simulink library "halout"  (R2021b)
settings: Solver=VariableStepAuto  StartTime=0.0  StopTime=10.0  RelTol=1e-3
undefined symbols (not defined in the file): C_TASK_5MS_S, KHAL_CAN1TxReq_flg, KHAL_CAN2TxReq_flg, KHAL_CAN3TxReq_flg, KHAL_CAN4TxReq_flg, KHAL_CAN5TxReq_flg, KHAL_CAN6TxReq_flg, KHAL_CAN7TxReq_flg, TRUE
libraries: FVT_lib x65, simulink x6
(part 2 of 6)

== system halout/HAL_OUT/CAN1/FD1_C50_0_0x18F00503 ==
  BSCP_outputs : Inport  OutDataTypeStr=Bus: BSCP_outputs
  BOUTP_outputs : Inport  Port=2  OutDataTypeStr=Bus: BOUTP_outputs
  ActDriveDirect : Subsystem
  Ground : Ground
  bus_creator : BusCreator  Inputs=1  OutDataTypeStr=Bus: DT_CAN1_SG_FD1_C50_0  NonVirtualBus=on
  FD1_C50_0 : Outport
  wires:
  BSCP_outputs/1 -> [BSCP_outputs]
  BOUTP_outputs/1 -> [BOUTP_outputs]
  [CAN1_ActDriveDirect] -> bus_creator/1  "CAN1_ActDriveDirect"
  bus_creator/1 -> FD1_C50_0/1
  ActDriveDirect/1(CAN1_ActDriveDirect) -> [CAN1_ActDriveDirect]
  Ground/1 -> ActDriveDirect/1(ActDriveDirect)

== system halout/HAL_OUT/CAN1/FD1_C50_1_0xCF00300 ==
  BSCP_outputs : Inport  OutDataTypeStr=Bus: BSCP_outputs
  BOUTP_outputs : Inport  Port=2  OutDataTypeStr=Bus: BOUTP_outputs
  AccPedal1LowSW : Subsystem
  AccPedalPos1 : Subsystem
  EEC2MSGCS : Subsystem
  EEC2MSGCnt : Subsystem
  Ground{,1..3} (4 alike) : Ground
  bus_creator : BusCreator  Inputs=4  OutDataTypeStr=Bus: DT_CAN1_SG_FD1_C50_1  NonVirtualBus=on
  FD1_C50_1 : Outport
  wires:
  BSCP_outputs/1 -> [BSCP_outputs]
  BOUTP_outputs/1 -> [BOUTP_outputs]
  [CAN1_AccPedal1LowSW] -> bus_creator/1  "CAN1_AccPedal1LowSW"
  [CAN1_AccPedalPos1] -> bus_creator/2  "CAN1_AccPedalPos1"
  [CAN1_EEC2MSGCS] -> bus_creator/3  "CAN1_EEC2MSGCS"
  [CAN1_EEC2MSGCnt] -> bus_creator/4  "CAN1_EEC2MSGCnt"
  bus_creator/1 -> FD1_C50_1/1
  AccPedal1LowSW/1(CAN1_AccPedal1LowSW) -> [CAN1_AccPedal1LowSW]
  AccPedalPos1/1(CAN1_AccPedalPos1) -> [CAN1_AccPedalPos1]
  EEC2MSGCS/1(CAN1_EEC2MSGCS) -> [CAN1_EEC2MSGCS]
  EEC2MSGCnt/1(CAN1_EEC2MSGCnt) -> [CAN1_EEC2MSGCnt]
  Ground/1 -> AccPedal1LowSW/1(AccPedal1LowSW)
  Ground1/1 -> AccPedalPos1/1(AccPedalPos1)
  Ground2/1 -> EEC2MSGCS/1(EEC2MSGCS)
  Ground3/1 -> EEC2MSGCnt/1(EEC2MSGCnt)

== system halout/HAL_OUT/CAN1/FD1_C80_0_0x18F00203 ==
  BSCP_outputs : Inport  OutDataTypeStr=Bus: BSCP_outputs
  BOUTP_outputs : Inport  Port=2  OutDataTypeStr=Bus: BOUTP_outputs
  DLEngaged : Subsystem
  ShiftPgs : Subsystem
  bus_creator : BusCreator  Inputs=2  OutDataTypeStr=Bus: DT_CAN1_SG_FD1_C80_0  NonVirtualBus=on
  bus_selector : BusSelector  OutputSignals=VOUTP_DrivelineRelease_enum
  bus_selector1 : BusSelector  OutputSignals=VOUTP_ETC1ShiftrPgs_enum
  FD1_C80_0 : Outport
  wires:
  BSCP_outputs/1 -> [BSCP_outputs]
  BOUTP_outputs/1 -> [BOUTP_outputs]
  [CAN1_DLEngaged] -> bus_creator/1  "CAN1_DLEngaged"
  [CAN1_ShiftPgs] -> bus_creator/2  "CAN1_ShiftPgs"
  bus_creator/1 -> FD1_C80_0/1
  DLEngaged/1(CAN1_DLEngaged) -> [CAN1_DLEngaged]
  ShiftPgs/1(CAN1_ShiftPgs) -> [CAN1_ShiftPgs]
  bus_selector/1 -> DLEngaged/1(DLEngaged)  "<VOUTP_DrivelineRelease_enum>"
  [BOUTP_outputs] -> bus_selector/1
  bus_selector1/1 -> ShiftPgs/1(ShiftPgs)  "<VOUTP_ETC1ShiftrPgs_enum>"
  [BOUTP_outputs] -> bus_selector1/1

== system halout/HAL_OUT/CAN1/FD1_CE100_0_0x18EBFFEF ==
  BSCP_outputs : Inport  OutDataTypeStr=Bus: BSCP_outputs
  BOUTP_outputs : Inport  Port=2  OutDataTypeStr=Bus: BOUTP_outputs
  CFGEM1DT0 : Subsystem
  CFGEM1DT1 : Subsystem
  CFGEM1DT2 : Subsystem
  CFGEM1DT3 : Subsystem
  CFGEM1DT4 : Subsystem
  CFGEM1DT5 : Subsystem
  CFGEM1DT6 : Subsystem
  CFGEM1DT7 : Subsystem
  bus_creator : BusCreator  Inputs=8  OutDataTypeStr=Bus: DT_CAN1_SG_FD1_CE100_0  NonVirtualBus=on
  bus_selector : BusSelector  OutputSignals=VOUTP_DTbyte0_raw
  bus_selector1 : BusSelector  OutputSignals=VOUTP_DTbyte1_raw
  bus_selector2 : BusSelector  OutputSignals=VOUTP_DTbyte2_raw
  bus_selector3 : BusSelector  OutputSignals=VOUTP_DTbyte3_raw
  bus_selector4 : BusSelector  OutputSignals=VOUTP_DTbyte4_raw
  bus_selector5 : BusSelector  OutputSignals=VOUTP_DTbyte5_raw
  bus_selector6 : BusSelector  OutputSignals=VOUTP_DTbyte6_raw
  bus_selector7 : BusSelector  OutputSignals=VOUTP_DTbyte7_raw
  FD1_CE100_0 : Outport
  wires:
  BSCP_outputs/1 -> [BSCP_outputs]
  BOUTP_outputs/1 -> [BOUTP_outputs]
  [CAN1_CFGEM1DT0] -> bus_creator/1  "CAN1_CFGEM1DT0"
  [CAN1_CFGEM1DT1] -> bus_creator/2  "CAN1_CFGEM1DT1"
  [CAN1_CFGEM1DT2] -> bus_creator/3  "CAN1_CFGEM1DT2"
  [CAN1_CFGEM1DT3] -> bus_creator/4  "CAN1_CFGEM1DT3"
  [CAN1_CFGEM1DT4] -> bus_creator/5  "CAN1_CFGEM1DT4"
  [CAN1_CFGEM1DT5] -> bus_creator/6  "CAN1_CFGEM1DT5"
  [CAN1_CFGEM1DT6] -> bus_creator/7  "CAN1_CFGEM1DT6"
  [CAN1_CFGEM1DT7] -> bus_creator/8  "CAN1_CFGEM1DT7"
  bus_creator/1 -> FD1_CE100_0/1
  CFGEM1DT0/1(CAN1_CFGEM1DT0) -> [CAN1_CFGEM1DT0]
  CFGEM1DT1/1(CAN1_CFGEM1DT1) -> [CAN1_CFGEM1DT1]
  CFGEM1DT2/1(CAN1_CFGEM1DT2) -> [CAN1_CFGEM1DT2]
  CFGEM1DT3/1(CAN1_CFGEM1DT3) -> [CAN1_CFGEM1DT3]
  CFGEM1DT4/1(CAN1_CFGEM1DT4) -> [CAN1_CFGEM1DT4]
  CFGEM1DT5/1(CAN1_CFGEM1DT5) -> [CAN1_CFGEM1DT5]
  CFGEM1DT6/1(CAN1_CFGEM1DT6) -> [CAN1_CFGEM1DT6]
  CFGEM1DT7/1(CAN1_CFGEM1DT7) -> [CAN1_CFGEM1DT7]
  bus_selector/1 -> CFGEM1DT0/1(CFGEM1DT0)  "<VOUTP_DTbyte0_raw>"
  [BOUTP_outputs] -> bus_selector/1
  bus_selector1/1 -> CFGEM1DT1/1(CFGEM1DT1)  "<VOUTP_DTbyte1_raw>"
  [BOUTP_outputs] -> bus_selector1/1
  bus_selector2/1 -> CFGEM1DT2/1(CFGEM1DT2)  "<VOUTP_DTbyte2_raw>"
  [BOUTP_outputs] -> bus_selector2/1
  bus_selector3/1 -> CFGEM1DT3/1(CFGEM1DT3)  "<VOUTP_DTbyte3_raw>"
  [BOUTP_outputs] -> bus_selector3/1
  bus_selector4/1 -> CFGEM1DT4/1(CFGEM1DT4)  "<VOUTP_DTbyte4_raw>"
  [BOUTP_outputs] -> bus_selector4/1
  bus_selector5/1 -> CFGEM1DT5/1(CFGEM1DT5)  "<VOUTP_DTbyte5_raw>"
  [BOUTP_outputs] -> bus_selector5/1
  bus_selector6/1 -> CFGEM1DT6/1(CFGEM1DT6)  "<VOUTP_DTbyte6_raw>"
  [BOUTP_outputs] -> bus_selector6/1
  bus_selector7/1 -> CFGEM1DT7/1(CFGEM1DT7)  "<VOUTP_DTbyte7_raw>"
  [BOUTP_outputs] -> bus_selector7/1

== system halout/HAL_OUT/CAN1/FD1_CE100_1_0x18ECFFEF ==
  BSCP_outputs : Inport  OutDataTypeStr=Bus: BSCP_outputs
  BOUTP_outputs : Inport  Port=2  OutDataTypeStr=Bus: BOUTP_outputs
  CFGEM1BAMPGN : Subsystem
  CFGEM1BAMRsv : Subsystem
  CFGEM1BAMTNum : Subsystem
  CFGEM1BAMTSize : Subsystem
  CFGEM1Ctrl : Subsystem
  bus_creator : BusCreator  Inputs=5  OutDataTypeStr=Bus: DT_CAN1_SG_FD1_CE100_1  NonVirtualBus=on
  bus_selector : BusSelector  OutputSignals=VOUTP_CFGEM1BAMPGN_raw
  bus_selector1 : BusSelector  OutputSignals=VOUTP_CFGEM1BAMRsv_raw
  bus_selector2 : BusSelector  OutputSignals=VOUTP_CFGEM1BAMTNum_raw
  bus_selector3 : BusSelector  OutputSignals=VOUTP_CFGEM1BAMTSize_raw
  bus_selector4 : BusSelector  OutputSignals=VOUTP_CFGEM1Ctrl_raw
  FD1_CE100_1 : Outport
  wires:
  BSCP_outputs/1 -> [BSCP_outputs]
  BOUTP_outputs/1 -> [BOUTP_outputs]
  [CAN1_CFGEM1BAMPGN] -> bus_creator/1  "CAN1_CFGEM1BAMPGN"
  [CAN1_CFGEM1BAMRsv] -> bus_creator/2  "CAN1_CFGEM1BAMRsv"
  [CAN1_CFGEM1BAMTNum] -> bus_creator/3  "CAN1_CFGEM1BAMTNum"
  [CAN1_CFGEM1BAMTSize] -> bus_creator/4  "CAN1_CFGEM1BAMTSize"
  [CAN1_CFGEM1Ctrl] -> bus_creator/5  "CAN1_CFGEM1Ctrl"
  bus_creator/1 -> FD1_CE100_1/1
  CFGEM1BAMPGN/1(CAN1_CFGEM1BAMPGN) -> [CAN1_CFGEM1BAMPGN]
  CFGEM1BAMRsv/1(CAN1_CFGEM1BAMRsv) -> [CAN1_CFGEM1BAMRsv]
  CFGEM1BAMTNum/1(CAN1_CFGEM1BAMTNum) -> [CAN1_CFGEM1BAMTNum]
  CFGEM1BAMTSize/1(CAN1_CFGEM1BAMTSize) -> [CAN1_CFGEM1BAMTSize]
  CFGEM1Ctrl/1(CAN1_CFGEM1Ctrl) -> [CAN1_CFGEM1Ctrl]
  bus_selector/1 -> CFGEM1BAMPGN/1(CFGEM1BAMPGN)  "<VOUTP_CFGEM1BAMPGN_raw>"
  [BOUTP_outputs] -> bus_selector/1
  bus_selector1/1 -> CFGEM1BAMRsv/1(CFGEM1BAMRsv)  "<VOUTP_CFGEM1BAMRsv_raw>"
  [BOUTP_outputs] -> bus_selector1/1
  bus_selector2/1 -> CFGEM1BAMTNum/1(CFGEM1BAMTNum)  "<VOUTP_CFGEM1BAMTNum_raw>"
  [BOUTP_outputs] -> bus_selector2/1
  bus_selector3/1 -> CFGEM1BAMTSize/1(CFGEM1BAMTSize)  "<VOUTP_CFGEM1BAMTSize_raw>"
  [BOUTP_outputs] -> bus_selector3/1
  bus_selector4/1 -> CFGEM1Ctrl/1(CFGEM1Ctrl)  "<VOUTP_CFGEM1Ctrl_raw>"
  [BOUTP_outputs] -> bus_selector4/1

== system halout/HAL_OUT/CAN1/FD1_CE100_2_0x18FA05B9 ==
  BSCP_outputs : Inport  OutDataTypeStr=Bus: BSCP_outputs
  BOUTP_outputs : Inport  Port=2  OutDataTypeStr=Bus: BOUTP_outputs
  FDCBCMDVRSignalLCmd : Subsystem
  FDCBCMDVRSignalRCmd : Subsystem
  FDCBCMLTurnLpCmd : Subsystem
  FDCBCMRTurnLpCmd : Subsystem
  bus_creator : BusCreator  Inputs=4  OutDataTypeStr=Bus: DT_CAN1_SG_FD1_CE100_2  NonVirtualBus=on
  bus_selector : BusSelector  OutputSignals=VOUTP_FDCBCMDVRSignalLCmd_flg
  bus_selector1 : BusSelector  OutputSignals=VOUTP_FDCBCMDVRSignalRCmd_flg
  bus_selector2 : BusSelector  OutputSignals=VOUTP_FDCBCMLTurnLpCmd_flg
  bus_selector3 : BusSelector  OutputSignals=VOUTP_FDCBCMRTurnLpCmd_flg
  FD1_CE100_2 : Outport
  wires:
  BSCP_outputs/1 -> [BSCP_outputs]
  BOUTP_outputs/1 -> [BOUTP_outputs]
  [CAN1_FDC_BCM_DVRSignalL_Cmd] -> bus_creator/1  "CAN1_FDC_BCM_DVRSignalL_Cmd"
  [CAN1_FDC_BCM_DVRSignalR_Cmd] -> bus_creator/2  "CAN1_FDC_BCM_DVRSignalR_Cmd"
  [CAN1_FDC_BCM_LTurnLp_Cmd] -> bus_creator/3  "CAN1_FDC_BCM_LTurnLp_Cmd"
  [CAN1_FDC_BCM_RTurnLp_Cmd] -> bus_creator/4  "CAN1_FDC_BCM_RTurnLp_Cmd"
  bus_creator/1 -> FD1_CE100_2/1
  FDCBCMDVRSignalLCmd/1(CAN1_FDC_BCM_DVRSignalL_Cmd) -> [CAN1_FDC_BCM_DVRSignalL_Cmd]
  FDCBCMDVRSignalRCmd/1(CAN1_FDC_BCM_DVRSignalR_Cmd) -> [CAN1_FDC_BCM_DVRSignalR_Cmd]
  FDCBCMLTurnLpCmd/1(CAN1_FDC_BCM_LTurnLp_Cmd) -> [CAN1_FDC_BCM_LTurnLp_Cmd]
  FDCBCMRTurnLpCmd/1(CAN1_FDC_BCM_RTurnLp_Cmd) -> [CAN1_FDC_BCM_RTurnLp_Cmd]
  bus_selector/1 -> FDCBCMDVRSignalLCmd/1(FDCBCMDVRSignalLCmd)  "<VOUTP_FDCBCMDVRSignalLCmd_flg>"
  [BOUTP_outputs] -> bus_selector/1
  bus_selector1/1 -> FDCBCMDVRSignalRCmd/1(FDCBCMDVRSignalRCmd)  "<VOUTP_FDCBCMDVRSignalRCmd_flg>"
  [BOUTP_outputs] -> bus_selector1/1
  bus_selector2/1 -> FDCBCMLTurnLpCmd/1(FDCBCMLTurnLpCmd)  "<VOUTP_FDCBCMLTurnLpCmd_flg>"
  [BOUTP_outputs] -> bus_selector2/1
  bus_selector3/1 -> FDCBCMRTurnLpCmd/1(FDCBCMRTurnLpCmd)  "<VOUTP_FDCBCMRTurnLpCmd_flg>"
  [BOUTP_outputs] -> bus_selector3/1

== system halout/HAL_OUT/CAN2/FD2_C1000_0_0x20E ==
  BSCP_outputs : Inport  OutDataTypeStr=Bus: BSCP_outputs
  BOUTP_outputs : Inport  Port=2  OutDataTypeStr=Bus: BOUTP_outputs
  VCUVehAcclLimit : Subsystem
  VCUVehSpdlimit : Subsystem
  bus_creator : BusCreator  Inputs=2  OutDataTypeStr=Bus: DT_CAN2_SG_FD2_C1000_0  NonVirtualBus=on
  bus_selector : BusSelector  OutputSignals=VOUTP_VehAcclLimitTG_mps2
  bus_selector1 : BusSelector  OutputSignals=VOUTP_VehSpdLimitTG_kph
  FD2_C1000_0 : Outport
  wires:
  BSCP_outputs/1 -> [BSCP_outputs]
  BOUTP_outputs/1 -> [BOUTP_outputs]
  [CAN2_VCUVehAcclLimit] -> bus_creator/1  "CAN2_VCUVehAcclLimit"
  [CAN2_VCUVehSpdlimit] -> bus_creator/2  "CAN2_VCUVehSpdlimit"
  bus_creator/1 -> FD2_C1000_0/1
  VCUVehAcclLimit/1(CAN2_VCUVehAcclLimit) -> [CAN2_VCUVehAcclLimit]
  VCUVehSpdlimit/1(CAN2_VCUVehSpdlimit) -> [CAN2_VCUVehSpdlimit]
  bus_selector/1 -> VCUVehAcclLimit/1(VCUVehAcclLimit)  "<VOUTP_VehAcclLimitTG_mps2>"
  [BOUTP_outputs] -> bus_selector/1
  bus_selector1/1 -> VCUVehSpdlimit/1(VCUVehSpdlimit)  "<VOUTP_VehSpdLimitTG_kph>"
  [BOUTP_outputs] -> bus_selector1/1

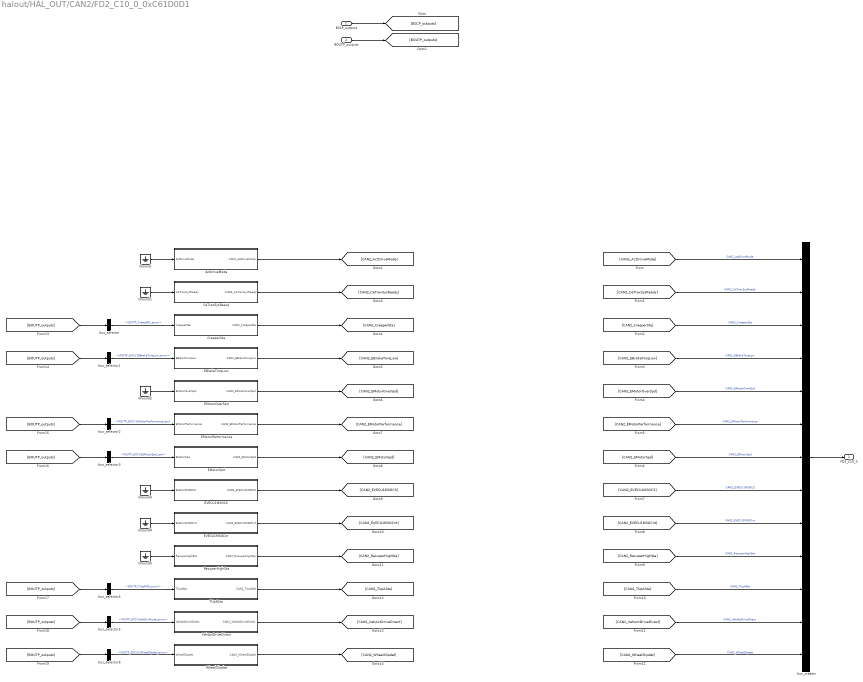
== system halout/HAL_OUT/CAN2/FD2_C10_0_0xC61D0D1 ==
  BSCP_outputs : Inport  OutDataTypeStr=Bus: BSCP_outputs
  BOUTP_outputs : Inport  Port=2  OutDataTypeStr=Bus: BOUTP_outputs
  ActDriveMode : Subsystem
  CeTraxSysReady : Subsystem
  CreeperSta : Subsystem
  EBrakeTorqLow : Subsystem
  EMotorOverSpd : Subsystem
  EMotorPerformance : Subsystem
  EMotorSpd : Subsystem
  EVECU1MSGCS : Subsystem
  EVECU1MSGCnt : Subsystem
  Ground{,1..5} (6 alike) : Ground
  RecuperHighSta : Subsystem
  TUpASta : Subsystem
  VehActDriveDirect : Subsystem
  WheelSlipdet : Subsystem
  bus_creator : BusCreator  Inputs=13  OutDataTypeStr=Bus: DT_CAN2_SG_FD2_C10_0  NonVirtualBus=on
  bus_selector : BusSelector  OutputSignals=VOUTP_CreepIND_enum
  bus_selector1 : BusSelector  OutputSignals=VOUTP_EVCU1EBrakeTorqLow_enum
  bus_selector2 : BusSelector  OutputSignals=VOUTP_EVCU1EMotorPerformance_pct
  bus_selector3 : BusSelector  OutputSignals=VOUTP_EVCU1EMotorSpd_rpm
  bus_selector4 : BusSelector  OutputSignals=VOUTP_TUpAIND_enum
  bus_selector5 : BusSelector  OutputSignals=VOUTP_EVCU1ActDrvMode_enum
  bus_selector6 : BusSelector  OutputSignals=VOUTP_EVCU1WheelSlipdet_enum
  FD2_C10_0 : Outport
  wires:
  BSCP_outputs/1 -> [BSCP_outputs]
  BOUTP_outputs/1 -> [BOUTP_outputs]
  [CAN2_ActDriveMode] -> bus_creator/1  "CAN2_ActDriveMode"
  [CAN2_CeTraxSysReady] -> bus_creator/2  "CAN2_CeTraxSysReady"
  [CAN2_CreeperSta] -> bus_creator/3  "CAN2_CreeperSta"
  [CAN2_EBrakeTorqLow] -> bus_creator/4  "CAN2_EBrakeTorqLow"
  [CAN2_EMotorOverSpd] -> bus_creator/5  "CAN2_EMotorOverSpd"
  [CAN2_EMotorPerformance] -> bus_creator/6  "CAN2_EMotorPerformance"
  [CAN2_EMotorSpd] -> bus_creator/7  "CAN2_EMotorSpd"
  [CAN2_EVECU1MSGCS] -> bus_creator/8  "CAN2_EVECU1MSGCS"
  [CAN2_EVECU1MSGCnt] -> bus_creator/9  "CAN2_EVECU1MSGCnt"
  [CAN2_RecuperHighSta] -> bus_creator/10  "CAN2_RecuperHighSta"
  [CAN2_TUpASta] -> bus_creator/11  "CAN2_TUpASta"
  [CAN2_VehActDriveDirect] -> bus_creator/12  "CAN2_VehActDriveDirect"
  [CAN2_WheelSlipdet] -> bus_creator/13  "CAN2_WheelSlipdet"
  bus_creator/1 -> FD2_C10_0/1
  ActDriveMode/1(CAN2_ActDriveMode) -> [CAN2_ActDriveMode]
  CeTraxSysReady/1(CAN2_CeTraxSysReady) -> [CAN2_CeTraxSysReady]
  CreeperSta/1(CAN2_CreeperSta) -> [CAN2_CreeperSta]
  EBrakeTorqLow/1(CAN2_EBrakeTorqLow) -> [CAN2_EBrakeTorqLow]
  EMotorOverSpd/1(CAN2_EMotorOverSpd) -> [CAN2_EMotorOverSpd]
  EMotorPerformance/1(CAN2_EMotorPerformance) -> [CAN2_EMotorPerformance]
  EMotorSpd/1(CAN2_EMotorSpd) -> [CAN2_EMotorSpd]
  EVECU1MSGCS/1(CAN2_EVECU1MSGCS) -> [CAN2_EVECU1MSGCS]
  EVECU1MSGCnt/1(CAN2_EVECU1MSGCnt) -> [CAN2_EVECU1MSGCnt]
  RecuperHighSta/1(CAN2_RecuperHighSta) -> [CAN2_RecuperHighSta]
  TUpASta/1(CAN2_TUpASta) -> [CAN2_TUpASta]
  VehActDriveDirect/1(CAN2_VehActDriveDirect) -> [CAN2_VehActDriveDirect]
  WheelSlipdet/1(CAN2_WheelSlipdet) -> [CAN2_WheelSlipdet]
  Ground/1 -> ActDriveMode/1(ActDriveMode)
  Ground1/1 -> CeTraxSysReady/1(CeTraxSysReady)
  bus_selector/1 -> CreeperSta/1(CreeperSta)  "<VOUTP_CreepIND_enum>"
  [BOUTP_outputs] -> bus_selector/1
  bus_selector1/1 -> EBrakeTorqLow/1(EBrakeTorqLow)  "<VOUTP_EVCU1EBrakeTorqLow_enum>"
  [BOUTP_outputs] -> bus_selector1/1
  Ground2/1 -> EMotorOverSpd/1(EMotorOverSpd)
  bus_selector2/1 -> EMotorPerformance/1(EMotorPerformance)  "<VOUTP_EVCU1EMotorPerformance_pct>"
  [BOUTP_outputs] -> bus_selector2/1
  bus_selector3/1 -> EMotorSpd/1(EMotorSpd)  "<VOUTP_EVCU1EMotorSpd_rpm>"
  [BOUTP_outputs] -> bus_selector3/1
  Ground3/1 -> EVECU1MSGCS/1(EVECU1MSGCS)
  Ground4/1 -> EVECU1MSGCnt/1(EVECU1MSGCnt)
  Ground5/1 -> RecuperHighSta/1(RecuperHighSta)
  bus_selector4/1 -> TUpASta/1(TUpASta)  "<VOUTP_TUpAIND_enum>"
  [BOUTP_outputs] -> bus_selector4/1
  bus_selector5/1 -> VehActDriveDirect/1(VehActDriveDirect)  "<VOUTP_EVCU1ActDrvMode_enum>"
  [BOUTP_outputs] -> bus_selector5/1
  bus_selector6/1 -> WheelSlipdet/1(WheelSlipdet)  "<VOUTP_EVCU1WheelSlipdet_enum>"
  [BOUTP_outputs] -> bus_selector6/1

== system halout/HAL_OUT/CAN2/FD2_C200_0_0x20F ==
  BSCP_outputs : Inport  OutDataTypeStr=Bus: BSCP_outputs
  BOUTP_outputs : Inport  Port=2  OutDataTypeStr=Bus: BOUTP_outputs
  CACPresWarn : Subsystem
  FDCVCUVCUDRMSta : Subsystem
  Ground : Ground
  SysPowerMode : Subsystem
  bus_creator : BusCreator  Inputs=3  OutDataTypeStr=Bus: DT_CAN2_SG_FD2_C200_0  NonVirtualBus=on
  bus_selector : BusSelector  OutputSignals=VOUTP_ActDriveMode_enum
  bus_selector1 : BusSelector  OutputSignals=VOUTP_SysPowerMode_enum
  FD2_C200_0 : Outport
  wires:
  BSCP_outputs/1 -> [BSCP_outputs]
  BOUTP_outputs/1 -> [BOUTP_outputs]
  [CAN2_CACPresWarn] -> bus_creator/1  "CAN2_CACPresWarn"
  [CAN2_FDC_VCU_VCUDRM_Sta] -> bus_creator/2  "CAN2_FDC_VCU_VCUDRM_Sta"
  [CAN2_SysPowerMode] -> bus_creator/3  "CAN2_SysPowerMode"
  bus_creator/1 -> FD2_C200_0/1
  CACPresWarn/1(CAN2_CACPresWarn) -> [CAN2_CACPresWarn]
  FDCVCUVCUDRMSta/1(CAN2_FDC_VCU_VCUDRM_Sta) -> [CAN2_FDC_VCU_VCUDRM_Sta]
  SysPowerMode/1(CAN2_SysPowerMode) -> [CAN2_SysPowerMode]
  Ground/1 -> CACPresWarn/1(CACPresWarn)
  bus_selector/1 -> FDCVCUVCUDRMSta/1(FDCVCUVCUDRMSta)  "<VOUTP_ActDriveMode_enum>"
  [BOUTP_outputs] -> bus_selector/1
  bus_selector1/1 -> SysPowerMode/1(SysPowerMode)  "<VOUTP_SysPowerMode_enum>"
  [BOUTP_outputs] -> bus_selector1/1

== system halout/HAL_OUT/CAN2/FD2_C500_0_0x18FA0517 ==
  BSCP_outputs : Inport  OutDataTypeStr=Bus: BSCP_outputs
  BOUTP_outputs : Inport  Port=2  OutDataTypeStr=Bus: BOUTP_outputs
  Ground : Ground
  IGNKeySta : Subsystem
  VCUVehicleSpd : Subsystem
  VSPFunc : Subsystem
  bus_creator : BusCreator  Inputs=3  OutDataTypeStr=Bus: DT_CAN2_SG_FD2_C500_0  NonVirtualBus=on
  bus_selector : BusSelector  OutputSignals=VOUTP_VSPIGNKeySta_enum
  bus_selector1 : BusSelector  OutputSignals=VOUTP_VCUTMVehSpd_kph
  FD2_C500_0 : Outport
  wires:
  BSCP_outputs/1 -> [BSCP_outputs]
  BOUTP_outputs/1 -> [BOUTP_outputs]
  [CAN2_IGNKeySta] -> bus_creator/1  "CAN2_IGNKeySta"
  [CAN2_VCU_VehicleSpd] -> bus_creator/2  "CAN2_VCU_VehicleSpd"
  [CAN2_VSPFunc] -> bus_creator/3  "CAN2_VSPFunc"
  bus_creator/1 -> FD2_C500_0/1
  IGNKeySta/1(CAN2_IGNKeySta) -> [CAN2_IGNKeySta]
  VCUVehicleSpd/1(CAN2_VCU_VehicleSpd) -> [CAN2_VCU_VehicleSpd]
  VSPFunc/1(CAN2_VSPFunc) -> [CAN2_VSPFunc]
  bus_selector/1 -> IGNKeySta/1(IGNKeySta)  "<VOUTP_VSPIGNKeySta_enum>"
  [BOUTP_outputs] -> bus_selector/1
  bus_selector1/1 -> VCUVehicleSpd/1(VCUVehicleSpd)  "<VOUTP_VCUTMVehSpd_kph>"
  [BOUTP_outputs] -> bus_selector1/1
  Ground/1 -> VSPFunc/1(VSPFunc)

== system halout/HAL_OUT/CAN2/FD2_C50_0_0xCFF355A ==
  BSCP_outputs : Inport  OutDataTypeStr=Bus: BSCP_outputs
  BOUTP_outputs : Inport  Port=2  OutDataTypeStr=Bus: BOUTP_outputs
  EVEHCMSGCS : Subsystem
  EVEHCMSGCnt : Subsystem
  EVSysRls : Subsystem
  ElecSysRdy : Subsystem
  ExtAccLimReq : Subsystem
  ExtDischgReq : Subsystem
  ExtDriveMReq : Subsystem
  ExtWorkshopMReq : Subsystem
  Ground{,1..5} (6 alike) : Ground
  RecuperLimOrReq : Subsystem
  bus_creator : BusCreator  Inputs=9  OutDataTypeStr=Bus: DT_CAN2_SG_FD2_C50_0  NonVirtualBus=on
  bus_selector : BusSelector  OutputSignals=VOUTP_DrivelineRelease_enum
  bus_selector1 : BusSelector  OutputSignals=VOUTP_HVSysReady_enum
  bus_selector2 : BusSelector  OutputSignals=VOUTP_ActiveDischargeReq_enum
  FD2_C50_0 : Outport
  wires:
  BSCP_outputs/1 -> [BSCP_outputs]
  BOUTP_outputs/1 -> [BOUTP_outputs]
  [CAN2_EVEHCMSGCS] -> bus_creator/1  "CAN2_EVEHCMSGCS"
  [CAN2_EVEHCMSGCnt] -> bus_creator/2  "CAN2_EVEHCMSGCnt"
  [CAN2_EVSysRls] -> bus_creator/3  "CAN2_EVSysRls"
  [CAN2_ElecSysRdy] -> bus_creator/4  "CAN2_ElecSysRdy"
  [CAN2_ExtAccLimReq] -> bus_creator/5  "CAN2_ExtAccLimReq"
  [CAN2_ExtDischgReq] -> bus_creator/6  "CAN2_ExtDischgReq"
  [CAN2_ExtDriveMReq] -> bus_creator/7  "CAN2_ExtDriveMReq"
  [CAN2_ExtWorkshopMReq] -> bus_creator/8  "CAN2_ExtWorkshopMReq"
  [CAN2_RecuperLimOrReq] -> bus_creator/9  "CAN2_RecuperLimOrReq"
  bus_creator/1 -> FD2_C50_0/1
  EVEHCMSGCS/1(CAN2_EVEHCMSGCS) -> [CAN2_EVEHCMSGCS]
  EVEHCMSGCnt/1(CAN2_EVEHCMSGCnt) -> [CAN2_EVEHCMSGCnt]
  EVSysRls/1(CAN2_EVSysRls) -> [CAN2_EVSysRls]
  ElecSysRdy/1(CAN2_ElecSysRdy) -> [CAN2_ElecSysRdy]
  ExtAccLimReq/1(CAN2_ExtAccLimReq) -> [CAN2_ExtAccLimReq]
  ExtDischgReq/1(CAN2_ExtDischgReq) -> [CAN2_ExtDischgReq]
  ExtDriveMReq/1(CAN2_ExtDriveMReq) -> [CAN2_ExtDriveMReq]
  ExtWorkshopMReq/1(CAN2_ExtWorkshopMReq) -> [CAN2_ExtWorkshopMReq]
  RecuperLimOrReq/1(CAN2_RecuperLimOrReq) -> [CAN2_RecuperLimOrReq]
  Ground/1 -> EVEHCMSGCS/1(EVEHCMSGCS)
  Ground1/1 -> EVEHCMSGCnt/1(EVEHCMSGCnt)
  bus_selector/1 -> EVSysRls/1(EVSysRls)  "<VOUTP_DrivelineRelease_enum>"
  [BOUTP_outputs] -> bus_selector/1
  bus_selector1/1 -> ElecSysRdy/1(ElecSysRdy)  "<VOUTP_HVSysReady_enum>"
  [BOUTP_outputs] -> bus_selector1/1
  Ground2/1 -> ExtAccLimReq/1(ExtAccLimReq)
  bus_selector2/1 -> ExtDischgReq/1(ExtDischgReq)  "<VOUTP_ActiveDischargeReq_enum>"
  [BOUTP_outputs] -> bus_selector2/1
  Ground3/1 -> ExtDriveMReq/1(ExtDriveMReq)
  Ground4/1 -> ExtWorkshopMReq/1(ExtWorkshopMReq)
  Ground5/1 -> RecuperLimOrReq/1(RecuperLimOrReq)

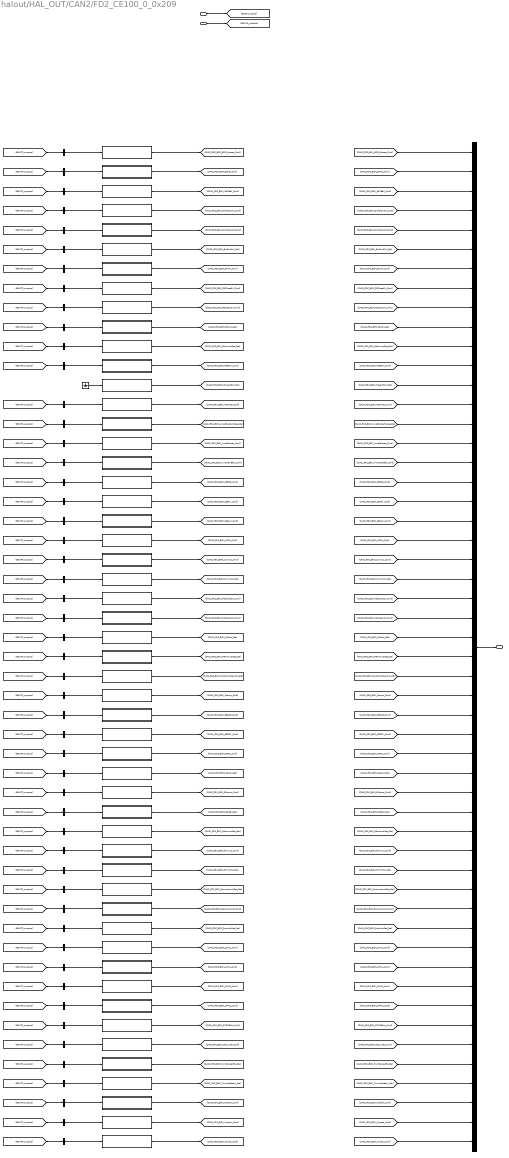
== system halout/HAL_OUT/CAN2/FD2_CE100_0_0x209 ==
  BSCP_outputs : Inport  OutDataTypeStr=Bus: BSCP_outputs
  BOUTP_outputs : Inport  Port=2  OutDataTypeStr=Bus: BOUTP_outputs
  FDCBCMBSDBuzzerCmd : Subsystem
  FDCBCMBrakeCmd : Subsystem
  FDCBCMCallBellCmd : Subsystem
  FDCBCMDVRSignalLCmd : Subsystem
  FDCBCMDVRSignalRCmd : Subsystem
  FDCBCMEmExitSWSta : Subsystem
  FDCBCMEmSVCmd : Subsystem
  FDCBCMFDCloseSVCmd : Subsystem
  FDCBCMFDOpenSVCmd : Subsystem
  FDCBCMFDoorSta : Subsystem
  FDCBCMFRoomLpSetSta : Subsystem
  FDCBCMHBeamCmd : Subsystem
  FDCBCMHazardSWSta : Subsystem
  FDCBCMHelpINDCmd : Subsystem
  FDCBCMInnerBuzzerCmd : Subsystem
  FDCBCMInnerBuzzerModeSta : Subsystem
  FDCBCMInnerCallBellCmd : Subsystem
  FDCBCMLBSDRCmd : Subsystem
  FDCBCMLBSDYCmd : Subsystem
  FDCBCMLBeamCmd : Subsystem
  FDCBCMLDRLCmd : Subsystem
  FDCBCMLTurnLpCmd : Subsystem
  FDCBCMLTurnSWSta : Subsystem
  FDCBCMMDCloseSVCmd : Subsystem
  FDCBCMMDOpenSVCmd : Subsystem
  FDCBCMMDoorSta : Subsystem
  FDCBCMMRoomLpSetSta : Subsystem
  FDCBCMOutDoorOpenSWSta : Subsystem
  FDCBCMPLampCmd : Subsystem
  FDCBCMRBSDRCmd : Subsystem
  FDCBCMRBSDYCmd : Subsystem
  FDCBCMRDRLCmd : Subsystem
  FDCBCMRDoorSta : Subsystem
  FDCBCMRFLampCmd : Subsystem
  FDCBCMRGearSta : Subsystem
  FDCBCMRRoomLpSetSta : Subsystem
  FDCBCMRTurnLpCmd : Subsystem
  FDCBCMRTurnSWSta : Subsystem
  FDCBCMRoomLpAmbCmd : Subsystem
  FDCBCMRoomLpAmbSetSta : Subsystem
  FDCBCMRoomLpSetSta : Subsystem
  FDCBCMSLTLpCmd : Subsystem
  FDCBCMSMKLCmd : Subsystem
  FDCBCMSMKRCmd : Subsystem
  FDCBCMSRTLpCmd : Subsystem
  FDCBCMSTOPBALLCmd : Subsystem
  FDCBCMStopINDCmd : Subsystem
  FDCBCMTurnBuzzerENSta : Subsystem
  FDCBCMTurnLpPatternSta : Subsystem
  FDCBCMWasherCmd : Subsystem
  FDCBCMWiperHCmd : Subsystem
  FDCBCMWiperLCmd : Subsystem
  Ground : Ground
  bus_creator : BusCreator  Inputs=52  OutDataTypeStr=Bus: DT_CAN2_SG_FD2_CE100_0  NonVirtualBus=on
  bus_selector : BusSelector  OutputSignals=VOUTP_FDCBCMBSDBuzzerCmd_flg
  bus_selector1 : BusSelector  OutputSignals=VOUTP_FDCBCMBrakeCmd_flg
  bus_selector10 : BusSelector  OutputSignals=VOUTP_FDCBCMFRoomLpSetSta_pct
  bus_selector11 : BusSelector  OutputSignals=VOUTP_FDCBCMHBeamCmd_flg
  bus_selector12 : BusSelector  OutputSignals=VOUTP_FDCBCMHelpINDCmd_flg
  bus_selector13 : BusSelector  OutputSignals=VOUTP_InnerBuzzerModeSta_enum
  bus_selector14 : BusSelector  OutputSignals=VOUTP_FDCBCMInnerBuzzerCmd_flg
  bus_selector15 : BusSelector  OutputSignals=VOUTP_FDCBCMInnerCallBellCmd_flg
  bus_selector16 : BusSelector  OutputSignals=VOUTP_FDCBCMLBSDRCmd_flg
  bus_selector17 : BusSelector  OutputSignals=VOUTP_FDCBCMLBSDYCmd_flg
  bus_selector18 : BusSelector  OutputSignals=VOUTP_FDCBCMLBeamCmd_flg
  bus_selector19 : BusSelector  OutputSignals=VOUTP_FDCBCMLDRLCmd_flg
  bus_selector2 : BusSelector  OutputSignals=VOUTP_FDCBCMCallBellCmd_flg
  bus_selector20 : BusSelector  OutputSignals=VOUTP_FDCBCMLTurnLpCmd_flg
  bus_selector21 : BusSelector  OutputSignals=VOUTP_FDCBCMLTurnSWSta_flg
  bus_selector22 : BusSelector  OutputSignals=VOUTP_FDCBCMMDCloseSVCmd_flg
  bus_selector23 : BusSelector  OutputSignals=VOUTP_FDCBCMMDOpenSVCmd_flg
  bus_selector24 : BusSelector  OutputSignals=VOUTP_FDCBCMMDoorSta_flg
  bus_selector25 : BusSelector  OutputSignals=VOUTP_FDCBCMMRoomLpSetSta_pct
  bus_selector26 : BusSelector  OutputSignals=VOUTP_FDCBCMOSDrOpenSWSta_enum
  bus_selector27 : BusSelector  OutputSignals=VOUTP_FDCBCMPLampCmd_flg
  bus_selector28 : BusSelector  OutputSignals=VOUTP_FDCBCMRBSDRCmd_flg
  bus_selector29 : BusSelector  OutputSignals=VOUTP_FDCBCMRBSDYCmd_flg
  bus_selector3 : BusSelector  OutputSignals=VOUTP_FDCBCMDVRSignalLCmd_flg
  bus_selector30 : BusSelector  OutputSignals=VOUTP_FDCBCMRDRLCmd_flg
  bus_selector31 : BusSelector  OutputSignals=VOUTP_FDCBCMRDoorSta_flg
  bus_selector32 : BusSelector  OutputSignals=VOUTP_FDCBCMRFLampCmd_flg
  bus_selector33 : BusSelector  OutputSignals=VOUTP_FDCBCMRGearSta_flg
  bus_selector34 : BusSelector  OutputSignals=VOUTP_FDCBCMRRoomLpSetSta_pct
  bus_selector35 : BusSelector  OutputSignals=VOUTP_FDCBCMRTurnLpCmd_flg
  bus_selector36 : BusSelector  OutputSignals=VOUTP_FDCBCMRTurnSWSta_flg
  bus_selector37 : BusSelector  OutputSignals=VOUTP_FDCBCMRoomLpAmbSetSta_flg
  bus_selector38 : BusSelector  OutputSignals=VOUTP_FDCBCMRoomLpAmbCmd_flg
  bus_selector39 : BusSelector  OutputSignals=VOUTP_FDCBCMRoomLpSetSta_flg
  bus_selector4 : BusSelector  OutputSignals=VOUTP_FDCBCMDVRSignalRCmd_flg
  bus_selector40 : BusSelector  OutputSignals=VOUTP_FDCBCMSLTLpCmd_flg
  bus_selector41 : BusSelector  OutputSignals=VOUTP_FDCBCMSMKLCmd_flg
  bus_selector42 : BusSelector  OutputSignals=VOUTP_FDCBCMSMKRCmd_flg
  bus_selector43 : BusSelector  OutputSignals=VOUTP_FDCBCMSRTLpCmd_flg
  bus_selector44 : BusSelector  OutputSignals=VOUTP_FDCBCMSTOPBALLCmd_flg
  bus_selector45 : BusSelector  OutputSignals=VOUTP_FDCBCMStopINDCmd_flg
  bus_selector46 : BusSelector  OutputSignals=VOUTP_FDCBCMTurnBuzzerENSta_flg
  bus_selector47 : BusSelector  OutputSignals=VOUTP_TurnLpPatternSta_enum
  bus_selector48 : BusSelector  OutputSignals=VOUTP_FDCBCMWasherCmd_flg
  bus_selector49 : BusSelector  OutputSignals=VOUTP_FDCBCMWiperHCmd_flg
  bus_selector5 : BusSelector  OutputSignals=VOUTP_FDCBCMEmExitSWSta_flg
  bus_selector50 : BusSelector  OutputSignals=VOUTP_FDCBCMWiperLCmd_flg
  bus_selector6 : BusSelector  OutputSignals=VOUTP_FDCBCMEmSVCmd_flg
  bus_selector7 : BusSelector  OutputSignals=VOUTP_FDCBCMFDCloseSVCmd_flg
  bus_selector8 : BusSelector  OutputSignals=VOUTP_FDCBCMFDOpenSVCmd_flg
  bus_selector9 : BusSelector  OutputSignals=VOUTP_FDCBCMFDoorSta_flg
  FD2_CE100_0 : Outport
  wires:
  BSCP_outputs/1 -> [BSCP_outputs]
  BOUTP_outputs/1 -> [BOUTP_outputs]
  [CAN2_FDC_BCM_BSD_Buzzer_Cmd] -> bus_creator/1  "CAN2_FDC_BCM_BSD_Buzzer_Cmd"
  [CAN2_FDC_BCM_Brake_Cmd] -> bus_creator/2  "CAN2_FDC_BCM_Brake_Cmd"
  [CAN2_FDC_BCM_CallBell_Cmd] -> bus_creator/3  "CAN2_FDC_BCM_CallBell_Cmd"
  [CAN2_FDC_BCM_DVRSignalL_Cmd] -> bus_creator/4  "CAN2_FDC_BCM_DVRSignalL_Cmd"
  [CAN2_FDC_BCM_DVRSignalR_Cmd] -> bus_creator/5  "CAN2_FDC_BCM_DVRSignalR_Cmd"
  [CAN2_FDC_BCM_EmExitSW_Sta] -> bus_creator/6  "CAN2_FDC_BCM_EmExitSW_Sta"
  [CAN2_FDC_BCM_EmSV_Cmd] -> bus_creator/7  "CAN2_FDC_BCM_EmSV_Cmd"
  [CAN2_FDC_BCM_FDCloseSV_Cmd] -> bus_creator/8  "CAN2_FDC_BCM_FDCloseSV_Cmd"
  [CAN2_FDC_BCM_FDOpenSV_Cmd] -> bus_creator/9  "CAN2_FDC_BCM_FDOpenSV_Cmd"
  [CAN2_FDC_BCM_FDoor_Sta] -> bus_creator/10  "CAN2_FDC_BCM_FDoor_Sta"
  [CAN2_FDC_BCM_FRoomLpSet_Sta] -> bus_creator/11  "CAN2_FDC_BCM_FRoomLpSet_Sta"
  [CAN2_FDC_BCM_HBeam_Cmd] -> bus_creator/12  "CAN2_FDC_BCM_HBeam_Cmd"
  [CAN2_FDC_BCM_HazardSW_Sta] -> bus_creator/13  "CAN2_FDC_BCM_HazardSW_Sta"
  [CAN2_FDC_BCM_HelpIND_Cmd] -> bus_creator/14  "CAN2_FDC_BCM_HelpIND_Cmd"
  [CAN2_FDC_BCM_InnerBuzzerMode_Sta] -> bus_creator/15  "CAN2_FDC_BCM_InnerBuzzerMode_Sta"
  [CAN2_FDC_BCM_InnerBuzzer_Cmd] -> bus_creator/16  "CAN2_FDC_BCM_InnerBuzzer_Cmd"
  [CAN2_FDC_BCM_InnerCallBell_Cmd] -> bus_creator/17  "CAN2_FDC_BCM_InnerCallBell_Cmd"
  [CAN2_FDC_BCM_LBSDR_Cmd] -> bus_creator/18  "CAN2_FDC_BCM_LBSDR_Cmd"
  [CAN2_FDC_BCM_LBSDY_Cmd] -> bus_creator/19  "CAN2_FDC_BCM_LBSDY_Cmd"
  [CAN2_FDC_BCM_LBeam_Cmd] -> bus_creator/20  "CAN2_FDC_BCM_LBeam_Cmd"
  [CAN2_FDC_BCM_LDRL_Cmd] -> bus_creator/21  "CAN2_FDC_BCM_LDRL_Cmd"
  [CAN2_FDC_BCM_LTurnLp_Cmd] -> bus_creator/22  "CAN2_FDC_BCM_LTurnLp_Cmd"
  [CAN2_FDC_BCM_LTurnSW_Sta] -> bus_creator/23  "CAN2_FDC_BCM_LTurnSW_Sta"
  [CAN2_FDC_BCM_MDCloseSV_Cmd] -> bus_creator/24  "CAN2_FDC_BCM_MDCloseSV_Cmd"
  [CAN2_FDC_BCM_MDOpenSV_Cmd] -> bus_creator/25  "CAN2_FDC_BCM_MDOpenSV_Cmd"
  [CAN2_FDC_BCM_MDoor_Sta] -> bus_creator/26  "CAN2_FDC_BCM_MDoor_Sta"
  [CAN2_FDC_BCM_MRoomLpSet_Sta] -> bus_creator/27  "CAN2_FDC_BCM_MRoomLpSet_Sta"
  [CAN2_FDC_BCM_OutDoorOpenSW_Sta] -> bus_creator/28  "CAN2_FDC_BCM_OutDoorOpenSW_Sta"
  [CAN2_FDC_BCM_PLamp_Cmd] -> bus_creator/29  "CAN2_FDC_BCM_PLamp_Cmd"
  [CAN2_FDC_BCM_RBSDR_Cmd] -> bus_creator/30  "CAN2_FDC_BCM_RBSDR_Cmd"
  [CAN2_FDC_BCM_RBSDY_Cmd] -> bus_creator/31  "CAN2_FDC_BCM_RBSDY_Cmd"
  [CAN2_FDC_BCM_RDRL_Cmd] -> bus_creator/32  "CAN2_FDC_BCM_RDRL_Cmd"
  [CAN2_FDC_BCM_RDoor_Sta] -> bus_creator/33  "CAN2_FDC_BCM_RDoor_Sta"
  [CAN2_FDC_BCM_RFLamp_Cmd] -> bus_creator/34  "CAN2_FDC_BCM_RFLamp_Cmd"
  [CAN2_FDC_BCM_RGear_Sta] -> bus_creator/35  "CAN2_FDC_BCM_RGear_Sta"
  [CAN2_FDC_BCM_RRoomLpSet_Sta] -> bus_creator/36  "CAN2_FDC_BCM_RRoomLpSet_Sta"
  [CAN2_FDC_BCM_RTurnLp_Cmd] -> bus_creator/37  "CAN2_FDC_BCM_RTurnLp_Cmd"
  [CAN2_FDC_BCM_RTurnSW_Sta] -> bus_creator/38  "CAN2_FDC_BCM_RTurnSW_Sta"
  [CAN2_FDC_BCM_RoomLpAmbSet_Sta] -> bus_creator/39  "CAN2_FDC_BCM_RoomLpAmbSet_Sta"
  [CAN2_FDC_BCM_RoomLpAmb_Cmd] -> bus_creator/40  "CAN2_FDC_BCM_RoomLpAmb_Cmd"
  [CAN2_FDC_BCM_RoomLpSet_Sta] -> bus_creator/41  "CAN2_FDC_BCM_RoomLpSet_Sta"
  [CAN2_FDC_BCM_SLTLp_Cmd] -> bus_creator/42  "CAN2_FDC_BCM_SLTLp_Cmd"
  [CAN2_FDC_BCM_SMKL_Cmd] -> bus_creator/43  "CAN2_FDC_BCM_SMKL_Cmd"
  [CAN2_FDC_BCM_SMKR_Cmd] -> bus_creator/44  "CAN2_FDC_BCM_SMKR_Cmd"
  [CAN2_FDC_BCM_SRTLp_Cmd] -> bus_creator/45  "CAN2_FDC_BCM_SRTLp_Cmd"
  [CAN2_FDC_BCM_STOPBALL_Cmd] -> bus_creator/46  "CAN2_FDC_BCM_STOPBALL_Cmd"
  [CAN2_FDC_BCM_Stop_IND_Cmd] -> bus_creator/47  "CAN2_FDC_BCM_Stop_IND_Cmd"
  [CAN2_FDC_BCM_TurnBuzzerEN_Sta] -> bus_creator/48  "CAN2_FDC_BCM_TurnBuzzerEN_Sta"
  [CAN2_FDC_BCM_TurnLpPattern_Sta] -> bus_creator/49  "CAN2_FDC_BCM_TurnLpPattern_Sta"
  [CAN2_FDC_BCM_Washer_Cmd] -> bus_creator/50  "CAN2_FDC_BCM_Washer_Cmd"
  [CAN2_FDC_BCM_WiperH_Cmd] -> bus_creator/51  "CAN2_FDC_BCM_WiperH_Cmd"
  [CAN2_FDC_BCM_WiperL_Cmd] -> bus_creator/52  "CAN2_FDC_BCM_WiperL_Cmd"
  bus_creator/1 -> FD2_CE100_0/1
  FDCBCMBSDBuzzerCmd/1(CAN2_FDC_BCM_BSD_Buzzer_Cmd) -> [CAN2_FDC_BCM_BSD_Buzzer_Cmd]
  FDCBCMBrakeCmd/1(CAN2_FDC_BCM_Brake_Cmd) -> [CAN2_FDC_BCM_Brake_Cmd]
  FDCBCMCallBellCmd/1(CAN2_FDC_BCM_CallBell_Cmd) -> [CAN2_FDC_BCM_CallBell_Cmd]
  FDCBCMDVRSignalLCmd/1(CAN2_FDC_BCM_DVRSignalL_Cmd) -> [CAN2_FDC_BCM_DVRSignalL_Cmd]
  FDCBCMDVRSignalRCmd/1(CAN2_FDC_BCM_DVRSignalR_Cmd) -> [CAN2_FDC_BCM_DVRSignalR_Cmd]
  FDCBCMEmExitSWSta/1(CAN2_FDC_BCM_EmExitSW_Sta) -> [CAN2_FDC_BCM_EmExitSW_Sta]
  FDCBCMEmSVCmd/1(CAN2_FDC_BCM_EmSV_Cmd) -> [CAN2_FDC_BCM_EmSV_Cmd]
  FDCBCMFDCloseSVCmd/1(CAN2_FDC_BCM_FDCloseSV_Cmd) -> [CAN2_FDC_BCM_FDCloseSV_Cmd]
  FDCBCMFDOpenSVCmd/1(CAN2_FDC_BCM_FDOpenSV_Cmd) -> [CAN2_FDC_BCM_FDOpenSV_Cmd]
  FDCBCMFDoorSta/1(CAN2_FDC_BCM_FDoor_Sta) -> [CAN2_FDC_BCM_FDoor_Sta]
  FDCBCMFRoomLpSetSta/1(CAN2_FDC_BCM_FRoomLpSet_Sta) -> [CAN2_FDC_BCM_FRoomLpSet_Sta]
  FDCBCMHBeamCmd/1(CAN2_FDC_BCM_HBeam_Cmd) -> [CAN2_FDC_BCM_HBeam_Cmd]
  FDCBCMHazardSWSta/1(CAN2_FDC_BCM_HazardSW_Sta) -> [CAN2_FDC_BCM_HazardSW_Sta]
  FDCBCMHelpINDCmd/1(CAN2_FDC_BCM_HelpIND_Cmd) -> [CAN2_FDC_BCM_HelpIND_Cmd]
  FDCBCMInnerBuzzerModeSta/1(CAN2_FDC_BCM_InnerBuzzerMode_Sta) -> [CAN2_FDC_BCM_InnerBuzzerMode_Sta]
  FDCBCMInnerBuzzerCmd/1(CAN2_FDC_BCM_InnerBuzzer_Cmd) -> [CAN2_FDC_BCM_InnerBuzzer_Cmd]
  FDCBCMInnerCallBellCmd/1(CAN2_FDC_BCM_InnerCallBell_Cmd) -> [CAN2_FDC_BCM_InnerCallBell_Cmd]
  FDCBCMLBSDRCmd/1(CAN2_FDC_BCM_LBSDR_Cmd) -> [CAN2_FDC_BCM_LBSDR_Cmd]
  FDCBCMLBSDYCmd/1(CAN2_FDC_BCM_LBSDY_Cmd) -> [CAN2_FDC_BCM_LBSDY_Cmd]
  FDCBCMLBeamCmd/1(CAN2_FDC_BCM_LBeam_Cmd) -> [CAN2_FDC_BCM_LBeam_Cmd]
  FDCBCMLDRLCmd/1(CAN2_FDC_BCM_LDRL_Cmd) -> [CAN2_FDC_BCM_LDRL_Cmd]
  FDCBCMLTurnLpCmd/1(CAN2_FDC_BCM_LTurnLp_Cmd) -> [CAN2_FDC_BCM_LTurnLp_Cmd]
  FDCBCMLTurnSWSta/1(CAN2_FDC_BCM_LTurnSW_Sta) -> [CAN2_FDC_BCM_LTurnSW_Sta]
  FDCBCMMDCloseSVCmd/1(CAN2_FDC_BCM_MDCloseSV_Cmd) -> [CAN2_FDC_BCM_MDCloseSV_Cmd]
  FDCBCMMDOpenSVCmd/1(CAN2_FDC_BCM_MDOpenSV_Cmd) -> [CAN2_FDC_BCM_MDOpenSV_Cmd]
  FDCBCMMDoorSta/1(CAN2_FDC_BCM_MDoor_Sta) -> [CAN2_FDC_BCM_MDoor_Sta]
  FDCBCMMRoomLpSetSta/1(CAN2_FDC_BCM_MRoomLpSet_Sta) -> [CAN2_FDC_BCM_MRoomLpSet_Sta]
  FDCBCMOutDoorOpenSWSta/1(CAN2_FDC_BCM_OutDoorOpenSW_Sta) -> [CAN2_FDC_BCM_OutDoorOpenSW_Sta]
  FDCBCMPLampCmd/1(CAN2_FDC_BCM_PLamp_Cmd) -> [CAN2_FDC_BCM_PLamp_Cmd]
  FDCBCMRBSDRCmd/1(CAN2_FDC_BCM_RBSDR_Cmd) -> [CAN2_FDC_BCM_RBSDR_Cmd]
  FDCBCMRBSDYCmd/1(CAN2_FDC_BCM_RBSDY_Cmd) -> [CAN2_FDC_BCM_RBSDY_Cmd]
  FDCBCMRDRLCmd/1(CAN2_FDC_BCM_RDRL_Cmd) -> [CAN2_FDC_BCM_RDRL_Cmd]
  FDCBCMRDoorSta/1(CAN2_FDC_BCM_RDoor_Sta) -> [CAN2_FDC_BCM_RDoor_Sta]
  FDCBCMRFLampCmd/1(CAN2_FDC_BCM_RFLamp_Cmd) -> [CAN2_FDC_BCM_RFLamp_Cmd]
  FDCBCMRGearSta/1(CAN2_FDC_BCM_RGear_Sta) -> [CAN2_FDC_BCM_RGear_Sta]
  FDCBCMRRoomLpSetSta/1(CAN2_FDC_BCM_RRoomLpSet_Sta) -> [CAN2_FDC_BCM_RRoomLpSet_Sta]
  FDCBCMRTurnLpCmd/1(CAN2_FDC_BCM_RTurnLp_Cmd) -> [CAN2_FDC_BCM_RTurnLp_Cmd]
  FDCBCMRTurnSWSta/1(CAN2_FDC_BCM_RTurnSW_Sta) -> [CAN2_FDC_BCM_RTurnSW_Sta]
  FDCBCMRoomLpAmbSetSta/1(CAN2_FDC_BCM_RoomLpAmbSet_Sta) -> [CAN2_FDC_BCM_RoomLpAmbSet_Sta]
  FDCBCMRoomLpAmbCmd/1(CAN2_FDC_BCM_RoomLpAmb_Cmd) -> [CAN2_FDC_BCM_RoomLpAmb_Cmd]
  FDCBCMRoomLpSetSta/1(CAN2_FDC_BCM_RoomLpSet_Sta) -> [CAN2_FDC_BCM_RoomLpSet_Sta]
  FDCBCMSLTLpCmd/1(CAN2_FDC_BCM_SLTLp_Cmd) -> [CAN2_FDC_BCM_SLTLp_Cmd]
  FDCBCMSMKLCmd/1(CAN2_FDC_BCM_SMKL_Cmd) -> [CAN2_FDC_BCM_SMKL_Cmd]
  FDCBCMSMKRCmd/1(CAN2_FDC_BCM_SMKR_Cmd) -> [CAN2_FDC_BCM_SMKR_Cmd]
  FDCBCMSRTLpCmd/1(CAN2_FDC_BCM_SRTLp_Cmd) -> [CAN2_FDC_BCM_SRTLp_Cmd]
  FDCBCMSTOPBALLCmd/1(CAN2_FDC_BCM_STOPBALL_Cmd) -> [CAN2_FDC_BCM_STOPBALL_Cmd]
  FDCBCMStopINDCmd/1(CAN2_FDC_BCM_Stop_IND_Cmd) -> [CAN2_FDC_BCM_Stop_IND_Cmd]
  FDCBCMTurnBuzzerENSta/1(CAN2_FDC_BCM_TurnBuzzerEN_Sta) -> [CAN2_FDC_BCM_TurnBuzzerEN_Sta]
  FDCBCMTurnLpPatternSta/1(CAN2_FDC_BCM_TurnLpPattern_Sta) -> [CAN2_FDC_BCM_TurnLpPattern_Sta]
  FDCBCMWasherCmd/1(CAN2_FDC_BCM_Washer_Cmd) -> [CAN2_FDC_BCM_Washer_Cmd]
  FDCBCMWiperHCmd/1(CAN2_FDC_BCM_WiperH_Cmd) -> [CAN2_FDC_BCM_WiperH_Cmd]
  FDCBCMWiperLCmd/1(CAN2_FDC_BCM_WiperL_Cmd) -> [CAN2_FDC_BCM_WiperL_Cmd]
  bus_selector/1 -> FDCBCMBSDBuzzerCmd/1(FDCBCMBSDBuzzerCmd)  "<VOUTP_FDCBCMBSDBuzzerCmd_flg>"
  [BOUTP_outputs] -> bus_selector/1
  bus_selector1/1 -> FDCBCMBrakeCmd/1(FDCBCMBrakeCmd)  "<VOUTP_FDCBCMBrakeCmd_flg>"
  [BOUTP_outputs] -> bus_selector1/1
  bus_selector2/1 -> FDCBCMCallBellCmd/1(FDCBCMCallBellCmd)  "<VOUTP_FDCBCMCallBellCmd_flg>"
  [BOUTP_outputs] -> bus_selector2/1
  bus_selector3/1 -> FDCBCMDVRSignalLCmd/1(FDCBCMDVRSignalLCmd)  "<VOUTP_FDCBCMDVRSignalLCmd_flg>"
  [BOUTP_outputs] -> bus_selector3/1
  bus_selector4/1 -> FDCBCMDVRSignalRCmd/1(FDCBCMDVRSignalRCmd)  "<VOUTP_FDCBCMDVRSignalRCmd_flg>"
  [BOUTP_outputs] -> bus_selector4/1
  bus_selector5/1 -> FDCBCMEmExitSWSta/1(FDCBCMEmExitSWSta)  "<VOUTP_FDCBCMEmExitSWSta_flg>"
  [BOUTP_outputs] -> bus_selector5/1
  bus_selector6/1 -> FDCBCMEmSVCmd/1(FDCBCMEmSVCmd)  "<VOUTP_FDCBCMEmSVCmd_flg>"
  [BOUTP_outputs] -> bus_selector6/1
  bus_selector7/1 -> FDCBCMFDCloseSVCmd/1(FDCBCMFDCloseSVCmd)  "<VOUTP_FDCBCMFDCloseSVCmd_flg>"
  [BOUTP_outputs] -> bus_selector7/1
  bus_selector8/1 -> FDCBCMFDOpenSVCmd/1(FDCBCMFDOpenSVCmd)  "<VOUTP_FDCBCMFDOpenSVCmd_flg>"
  [BOUTP_outputs] -> bus_selector8/1
  bus_selector9/1 -> FDCBCMFDoorSta/1(FDCBCMFDoorSta)  "<VOUTP_FDCBCMFDoorSta_flg>"
  [BOUTP_outputs] -> bus_selector9/1
  bus_selector10/1 -> FDCBCMFRoomLpSetSta/1(FDCBCMFRoomLpSetSta)  "<VOUTP_FDCBCMFRoomLpSetSta_pct>"
  [BOUTP_outputs] -> bus_selector10/1
  bus_selector11/1 -> FDCBCMHBeamCmd/1(FDCBCMHBeamCmd)  "<VOUTP_FDCBCMHBeamCmd_flg>"
  [BOUTP_outputs] -> bus_selector11/1
  Ground/1 -> FDCBCMHazardSWSta/1(FDCBCMHazardSWSta)
  bus_selector12/1 -> FDCBCMHelpINDCmd/1(FDCBCMHelpINDCmd)  "<VOUTP_FDCBCMHelpINDCmd_flg>"
  [BOUTP_outputs] -> bus_selector12/1
  bus_selector13/1 -> FDCBCMInnerBuzzerModeSta/1(FDCBCMInnerBuzzerModeSta)  "<VOUTP_InnerBuzzerModeSta_enum>"
  [BOUTP_outputs] -> bus_selector13/1
  bus_selector14/1 -> FDCBCMInnerBuzzerCmd/1(FDCBCMInnerBuzzerCmd)  "<VOUTP_FDCBCMInnerBuzzerCmd_flg>"
  [BOUTP_outputs] -> bus_selector14/1
  bus_selector15/1 -> FDCBCMInnerCallBellCmd/1(FDCBCMInnerCallBellCmd)  "<VOUTP_FDCBCMInnerCallBellCmd_flg>"
  [BOUTP_outputs] -> bus_selector15/1
  bus_selector16/1 -> FDCBCMLBSDRCmd/1(FDCBCMLBSDRCmd)  "<VOUTP_FDCBCMLBSDRCmd_flg>"
  [BOUTP_outputs] -> bus_selector16/1
  bus_selector17/1 -> FDCBCMLBSDYCmd/1(FDCBCMLBSDYCmd)  "<VOUTP_FDCBCMLBSDYCmd_flg>"
  [BOUTP_outputs] -> bus_selector17/1
  bus_selector18/1 -> FDCBCMLBeamCmd/1(FDCBCMLBeamCmd)  "<VOUTP_FDCBCMLBeamCmd_flg>"
  [BOUTP_outputs] -> bus_selector18/1
  bus_selector19/1 -> FDCBCMLDRLCmd/1(FDCBCMLDRLCmd)  "<VOUTP_FDCBCMLDRLCmd_flg>"
  [BOUTP_outputs] -> bus_selector19/1
  bus_selector20/1 -> FDCBCMLTurnLpCmd/1(FDCBCMLTurnLpCmd)  "<VOUTP_FDCBCMLTurnLpCmd_flg>"
  [BOUTP_outputs] -> bus_selector20/1
  bus_selector21/1 -> FDCBCMLTurnSWSta/1(FDCBCMLTurnSWSta)  "<VOUTP_FDCBCMLTurnSWSta_flg>"
  [BOUTP_outputs] -> bus_selector21/1
  bus_selector22/1 -> FDCBCMMDCloseSVCmd/1(FDCBCMMDCloseSVCmd)  "<VOUTP_FDCBCMMDCloseSVCmd_flg>"
  [BOUTP_outputs] -> bus_selector22/1
  bus_selector23/1 -> FDCBCMMDOpenSVCmd/1(FDCBCMMDOpenSVCmd)  "<VOUTP_FDCBCMMDOpenSVCmd_flg>"
  [BOUTP_outputs] -> bus_selector23/1
  bus_selector24/1 -> FDCBCMMDoorSta/1(FDCBCMMDoorSta)  "<VOUTP_FDCBCMMDoorSta_flg>"
  [BOUTP_outputs] -> bus_selector24/1
  bus_selector25/1 -> FDCBCMMRoomLpSetSta/1(FDCBCMMRoomLpSetSta)  "<VOUTP_FDCBCMMRoomLpSetSta_pct>"
  [BOUTP_outputs] -> bus_selector25/1
  bus_selector26/1 -> FDCBCMOutDoorOpenSWSta/1(FDCBCMOutDoorOpenSWSta)  "<VOUTP_FDCBCMOSDrOpenSWSta_enum>"
  [BOUTP_outputs] -> bus_selector26/1
  bus_selector27/1 -> FDCBCMPLampCmd/1(FDCBCMPLampCmd)  "<VOUTP_FDCBCMPLampCmd_flg>"
  [BOUTP_outputs] -> bus_selector27/1
  bus_selector28/1 -> FDCBCMRBSDRCmd/1(FDCBCMRBSDRCmd)  "<VOUTP_FDCBCMRBSDRCmd_flg>"
  [BOUTP_outputs] -> bus_selector28/1
  bus_selector29/1 -> FDCBCMRBSDYCmd/1(FDCBCMRBSDYCmd)  "<VOUTP_FDCBCMRBSDYCmd_flg>"
  [BOUTP_outputs] -> bus_selector29/1
  bus_selector30/1 -> FDCBCMRDRLCmd/1(FDCBCMRDRLCmd)  "<VOUTP_FDCBCMRDRLCmd_flg>"
  [BOUTP_outputs] -> bus_selector30/1
  bus_selector31/1 -> FDCBCMRDoorSta/1(FDCBCMRDoorSta)  "<VOUTP_FDCBCMRDoorSta_flg>"
  [BOUTP_outputs] -> bus_selector31/1
  bus_selector32/1 -> FDCBCMRFLampCmd/1(FDCBCMRFLampCmd)  "<VOUTP_FDCBCMRFLampCmd_flg>"
  [BOUTP_outputs] -> bus_selector32/1
  bus_selector33/1 -> FDCBCMRGearSta/1(FDCBCMRGearSta)  "<VOUTP_FDCBCMRGearSta_flg>"
  [BOUTP_outputs] -> bus_selector33/1
  bus_selector34/1 -> FDCBCMRRoomLpSetSta/1(FDCBCMRRoomLpSetSta)  "<VOUTP_FDCBCMRRoomLpSetSta_pct>"
  [BOUTP_outputs] -> bus_selector34/1
  bus_selector35/1 -> FDCBCMRTurnLpCmd/1(FDCBCMRTurnLpCmd)  "<VOUTP_FDCBCMRTurnLpCmd_flg>"
  [BOUTP_outputs] -> bus_selector35/1
  bus_selector36/1 -> FDCBCMRTurnSWSta/1(FDCBCMRTurnSWSta)  "<VOUTP_FDCBCMRTurnSWSta_flg>"
  [BOUTP_outputs] -> bus_selector36/1
  bus_selector37/1 -> FDCBCMRoomLpAmbSetSta/1(FDCBCMRoomLpAmbSetSta)  "<VOUTP_FDCBCMRoomLpAmbSetSta_flg>"
  [BOUTP_outputs] -> bus_selector37/1
  bus_selector38/1 -> FDCBCMRoomLpAmbCmd/1(FDCBCMRoomLpAmbCmd)  "<VOUTP_FDCBCMRoomLpAmbCmd_flg>"
  [BOUTP_outputs] -> bus_selector38/1
  bus_selector39/1 -> FDCBCMRoomLpSetSta/1(FDCBCMRoomLpSetSta)  "<VOUTP_FDCBCMRoomLpSetSta_flg>"
  [BOUTP_outputs] -> bus_selector39/1
  bus_selector40/1 -> FDCBCMSLTLpCmd/1(FDCBCMSLTLpCmd)  "<VOUTP_FDCBCMSLTLpCmd_flg>"
  [BOUTP_outputs] -> bus_selector40/1
  bus_selector41/1 -> FDCBCMSMKLCmd/1(FDCBCMSMKLCmd)  "<VOUTP_FDCBCMSMKLCmd_flg>"
  [BOUTP_outputs] -> bus_selector41/1
  bus_selector42/1 -> FDCBCMSMKRCmd/1(FDCBCMSMKRCmd)  "<VOUTP_FDCBCMSMKRCmd_flg>"
  [BOUTP_outputs] -> bus_selector42/1
  bus_selector43/1 -> FDCBCMSRTLpCmd/1(FDCBCMSRTLpCmd)  "<VOUTP_FDCBCMSRTLpCmd_flg>"
  [BOUTP_outputs] -> bus_selector43/1
  bus_selector44/1 -> FDCBCMSTOPBALLCmd/1(FDCBCMSTOPBALLCmd)  "<VOUTP_FDCBCMSTOPBALLCmd_flg>"
  [BOUTP_outputs] -> bus_selector44/1
  bus_selector45/1 -> FDCBCMStopINDCmd/1(FDCBCMStopINDCmd)  "<VOUTP_FDCBCMStopINDCmd_flg>"
  [BOUTP_outputs] -> bus_selector45/1
  bus_selector46/1 -> FDCBCMTurnBuzzerENSta/1(FDCBCMTurnBuzzerENSta)  "<VOUTP_FDCBCMTurnBuzzerENSta_flg>"
  [BOUTP_outputs] -> bus_selector46/1
  bus_selector47/1 -> FDCBCMTurnLpPatternSta/1(FDCBCMTurnLpPatternSta)  "<VOUTP_TurnLpPatternSta_enum>"
  [BOUTP_outputs] -> bus_selector47/1
  bus_selector48/1 -> FDCBCMWasherCmd/1(FDCBCMWasherCmd)  "<VOUTP_FDCBCMWasherCmd_flg>"
  [BOUTP_outputs] -> bus_selector48/1
  bus_selector49/1 -> FDCBCMWiperHCmd/1(FDCBCMWiperHCmd)  "<VOUTP_FDCBCMWiperHCmd_flg>"
  [BOUTP_outputs] -> bus_selector49/1
  bus_selector50/1 -> FDCBCMWiperLCmd/1(FDCBCMWiperLCmd)  "<VOUTP_FDCBCMWiperLCmd_flg>"
  [BOUTP_outputs] -> bus_selector50/1

== system halout/HAL_OUT/CAN2/GW2_C100_0_0x20B ==
  BSCP_outputs : Inport  OutDataTypeStr=Bus: BSCP_outputs
  BOUTP_outputs : Inport  Port=2  OutDataTypeStr=Bus: BOUTP_outputs
  CACTempWarn : Subsystem
  DACStatus : Subsystem
  GearFlashInd : Subsystem
  Ground : Ground
  Ground1 : Ground
  Ground2 : Ground
  LVBattLow : Subsystem
  PweLmtInd : Subsystem
  VCUWarnInd : Subsystem
  VCUnoPBInd : Subsystem
  bus_creator : BusCreator  Inputs=7  OutDataTypeStr=Bus: DT_CAN2_SG_GW2_C100_0  NonVirtualBus=on
  bus_selector : BusSelector  OutputSignals=VOUTP_GearFlashInd_flg
  bus_selector1 : BusSelector  OutputSignals=VOUTP_LVBattLowInd_enum
  bus_selector2 : BusSelector  OutputSignals=VOUTP_VCU4PweLmtInd_flg
  bus_selector3 : BusSelector  OutputSignals=VOUTP_ParkingProtectWarning_flg
  GW2_C100_0 : Outport
  wires:
  BSCP_outputs/1 -> [BSCP_outputs]
  BOUTP_outputs/1 -> [BOUTP_outputs]
  [CAN2_CACTempWarn] -> bus_creator/1  "CAN2_CACTempWarn"
  [CAN2_DACStatus] -> bus_creator/2  "CAN2_DACStatus"
  [CAN2_GearFlashInd] -> bus_creator/3  "CAN2_GearFlashInd"
  [CAN2_LVBattLow] -> bus_creator/4  "CAN2_LVBattLow"
  [CAN2_PweLmtInd] -> bus_creator/5  "CAN2_PweLmtInd"
  [CAN2_VCUWarnInd] -> bus_creator/6  "CAN2_VCUWarnInd"
  [CAN2_VCUnoPBInd] -> bus_creator/7  "CAN2_VCUnoPBInd"
  bus_creator/1 -> GW2_C100_0/1
  CACTempWarn/1(CAN2_CACTempWarn) -> [CAN2_CACTempWarn]
  DACStatus/1(CAN2_DACStatus) -> [CAN2_DACStatus]
  GearFlashInd/1(CAN2_GearFlashInd) -> [CAN2_GearFlashInd]
  LVBattLow/1(CAN2_LVBattLow) -> [CAN2_LVBattLow]
  PweLmtInd/1(CAN2_PweLmtInd) -> [CAN2_PweLmtInd]
  VCUWarnInd/1(CAN2_VCUWarnInd) -> [CAN2_VCUWarnInd]
  VCUnoPBInd/1(CAN2_VCUnoPBInd) -> [CAN2_VCUnoPBInd]
  Ground/1 -> CACTempWarn/1(CACTempWarn)
  Ground1/1 -> DACStatus/1(DACStatus)
  bus_selector/1 -> GearFlashInd/1(GearFlashInd)  "<VOUTP_GearFlashInd_flg>"
  [BOUTP_outputs] -> bus_selector/1
  bus_selector1/1 -> LVBattLow/1(LVBattLow)  "<VOUTP_LVBattLowInd_enum>"
  [BOUTP_outputs] -> bus_selector1/1
  bus_selector2/1 -> PweLmtInd/1(PweLmtInd)  "<VOUTP_VCU4PweLmtInd_flg>"
  [BOUTP_outputs] -> bus_selector2/1
  Ground2/1 -> VCUWarnInd/1(VCUWarnInd)
  bus_selector3/1 -> VCUnoPBInd/1(VCUnoPBInd)  "<VOUTP_ParkingProtectWarning_flg>"
  [BOUTP_outputs] -> bus_selector3/1
